simulink model "Pendulum_Motion_Simulation"  (R2020a)
settings: Solver=VariableStepAuto  StartTime=0.0  StopTime=20  MaxStep=1e-3  RelTol=1e-3
settings Model: Creator=Administrator  LastModifiedBy=Administrator

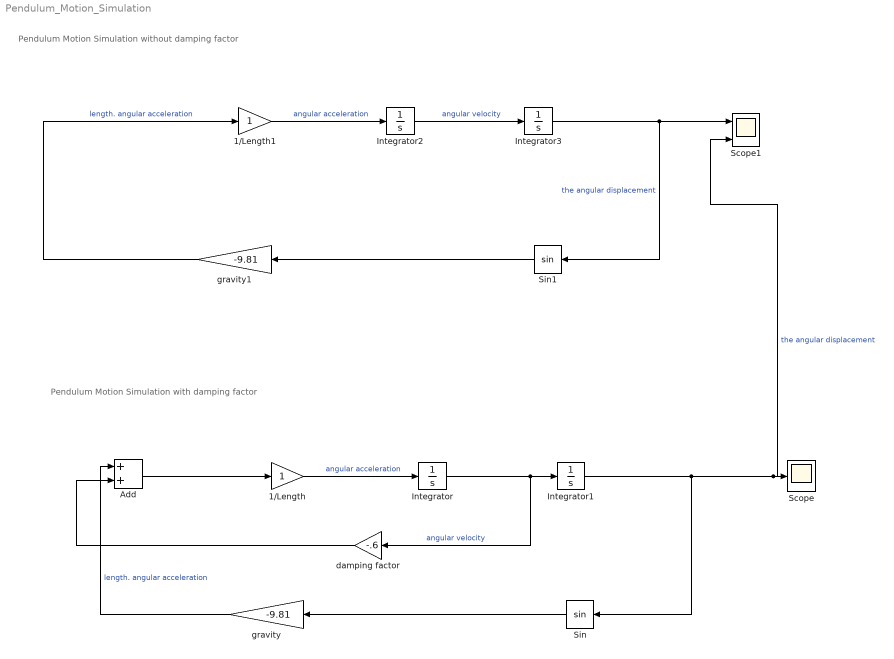
== system Pendulum_Motion_Simulation ==
  note: Pendulum Motion Simulation with damping factor
  note: Pendulum Motion Simulation without damping factor
  1/Length : Gain
  1/Length1 : Gain
  Add : Sum
  Integrator : Integrator
  Integrator1 : Integrator  InitialCondition=1
  Integrator2 : Integrator
  Integrator3 : Integrator  InitialCondition=1
  Scope : Scope
  Scope1 : Scope  NumInputPorts=2
  Sin : Trigonometry
  Sin1 : Trigonometry
  damping factor : Gain  Gain=-.6
  gravity : Gain  Gain=-9.81
  gravity1 : Gain  Gain=-9.81
  wires:
  Integrator/1 -> damping factor/1, Integrator1/1  "angular velocity"
  gravity/1 -> Add/1  "length. angular acceleration"
  Sin/1 -> gravity/1
  Integrator1/1 -> Sin/1, Scope1/2, Scope/1  "the angular displacement"
  1/Length/1 -> Integrator/1  "angular acceleration"
  Add/1 -> 1/Length/1
  damping factor/1 -> Add/2
  1/Length1/1 -> Integrator2/1  "angular acceleration"
  Integrator3/1 -> Sin1/1, Scope1/1  "the angular displacement"
  Sin1/1 -> gravity1/1
  gravity1/1 -> 1/Length1/1  "length. angular acceleration"
  Integrator2/1 -> Integrator3/1  "angular velocity"
